simulink library "mttlib"  (R2023a)
settings: Solver=VariableStepAuto  StartTime=0.0  StopTime=10.0  RelTol=1e-3
libraries: simulink x37, etargetslib x17, instrumentseriallib x2
settings Model: Creator=chrismailer  LastModifiedBy=JesseJabezArendse
settings ModelReferenceCC: EnableRefExpFcnMdlSchedulingChecks=on

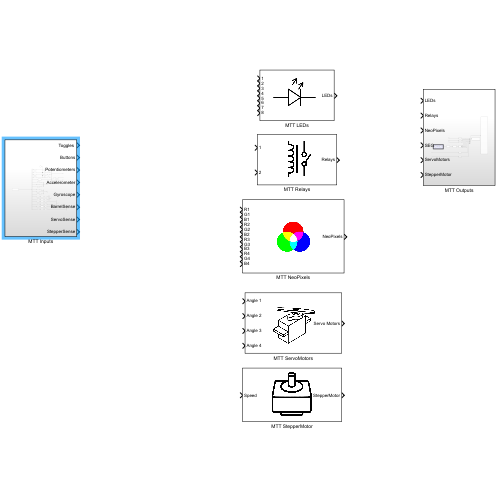
[thumbnail: Simulink's stored preview of the top-level diagram]
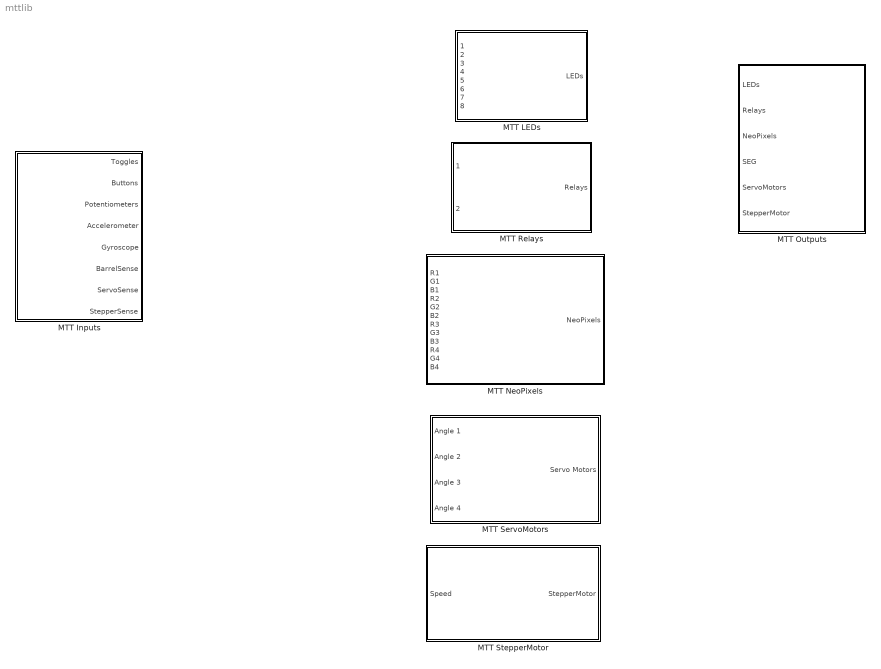
== system mttlib ==
  MTT Inputs : Subsystem
  MTT LEDs : Subsystem
      mask DialogControl DescGroupVar Prompt: MTT LEDs
      mask DialogControl DescTextVar Prompt: Initializing block for using the LEDs on the MTT board.
      mask Display: image('$imagefile'); % Use "Edit Image" on toolstrip to change.
  MTT NeoPixels : Subsystem
      mask DialogControl DescGroupVar Prompt: MTT NeoPixels
      mask DialogControl DescTextVar Prompt: Initializing block for using the NeoPixels on the MTT board.
      mask DialogControl Control2 Prompt: NeoPixels will not shine brigher when using values above 255, the brightness of each colour has been limited for eye comfort.
      mask Display: image('$imagefile'); % Use "Edit Image" on toolstrip to change.
  MTT Outputs : Subsystem
  MTT Relays : Subsystem
      mask DialogControl Container1 Prompt: MTT Relays
      mask DialogControl Control1 Prompt: Initializing block for the Relays on the MTT board.
      mask Display: image('$imagefile'); % Use "Edit Image" on toolstrip to change.
  MTT ServoMotors : Subsystem  mask{maxAngle1=0, startingTime1=0, maxAngle2=0, startingTime2=0, maxAngle3=0, startingTime3=0, maxAngle4=0, startingTime4=0}
      mask prompts: maxAngle1 "Max Angle (°):"; startingTime1 "Starting Time (μs):"; maxAngle2 "Max Angle (°):"; startingTime2 "Starting Time (μs):"; maxAngle3 "Max Angle (°):"; startingTime3 "Starting Time (μs):"; maxAngle4 "Max Angle (°):"; startingTime4 "Starting Time (μs):"
      mask DialogControl DescGroupVar Prompt: MTT ServoMotors
      mask DialogControl DescTextVar Prompt: Initializing block to use Servo Motors with MTT Board.
      mask DialogControl Control2 Prompt: Make sure to use non-zero values for servo parameters, they will not function otherwise.
      mask DialogControl Container1 Prompt: ServoMotor 1
      mask DialogControl Container2 Prompt: ServoMotor 2
      mask DialogControl Container3 Prompt: ServoMotor 3
      mask DialogControl Container4 Prompt: ServoMotor 4
      mask Display: image('$imagefile'); % Use "Edit Image" on toolstrip to change.
  MTT StepperMotor : Subsystem  mask{stepperMode=Full, stepperRevolution=1024}
      mask prompts: stepperMode "Mode:"; stepperRevolution "No. of steps for revolution:"
      mask TypeOptions stepperMode: Full | Wave | Half
      mask DialogControl DescGroupVar Prompt: MTT StepperMotor
      mask DialogControl DescTextVar Prompt: Initializing block for using a Stepper Motor on the MTT board.
      mask Display: image('$imagefile'); % Use "Edit Image" on toolstrip to change.

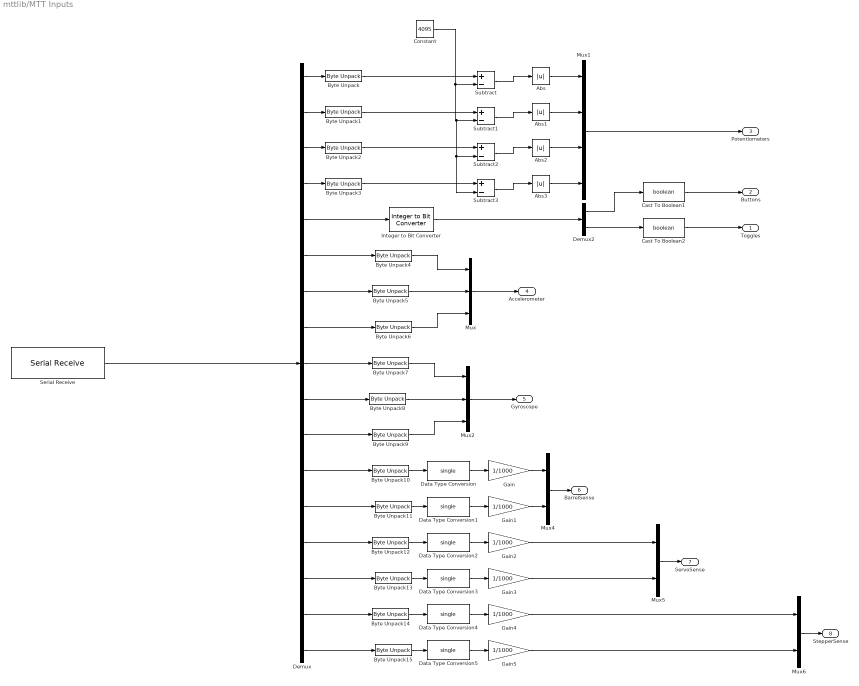
== system mttlib/MTT Inputs ==
  Abs{,1..3} (4 alike) : Abs  SaturateOnIntegerOverflow=off
  Byte Unpack{,1..3} (4 alike) : etargetslib/Byte Unpack  dimensions={[1]}  datatypes={'uint16'}  byteAlign=1
  Byte Unpack{10..15} (6 alike) : etargetslib/Byte Unpack  dimensions={[1]}  datatypes={'int16'}  byteAlign=1
  Byte Unpack{4..9} (6 alike) : etargetslib/Byte Unpack  dimensions={[1]}  datatypes={'single'}  byteAlign=1
  Cast To Boolean1 : DataTypeConversion  OutDataTypeStr=boolean  SaturateOnIntegerOverflow=off  RndMeth=Floor
  Cast To Boolean2 : DataTypeConversion  OutDataTypeStr=boolean  SaturateOnIntegerOverflow=off  RndMeth=Floor
  Constant : Constant  Value=4095
  Data Type Conversion{,1..5} (6 alike) : DataTypeConversion  OutDataTypeStr=single  SaturateOnIntegerOverflow=off  RndMeth=Floor
  Demux : Demux  Outputs=[2,2,2,2,1,4,4,4,4,4,4,2,2,2,2,2,2]
  Demux2 : Demux  Outputs=2
  Gain{,1..5} (6 alike) : Gain  Gain=1/1000
  Integer to Bit Converter : simulink/Logic and Bit Operations/Integer to Bit Converter  nbits=8  signedInputValues=Unsigned  bitOrder=MSB first  outDtype=boolean
  Mux : Mux  Inputs=3
  Mux1 : Mux
  Mux2 : Mux  Inputs=3
  Mux4 : Mux  Inputs=2
  Mux5 : Mux  Inputs=2
  Mux6 : Mux  Inputs=2
  Serial Receive : instrumentseriallib/Serial Receive  Priority=1  PortSel=COM17  Port=COM17  ComPort=COM17  DataType=uint8  SaveDataType=uint8  ToggleHeader=on  Header=0b10010010  ToggleTerminator=off  Terminator=<none>  CustomTerminator=[]  InputFormat=Column major  ToggleDataSize=on  DataSize=[1 45]  EnableBlockingMode=on  ActionDataUnavailable=Output last received value  ActionWhenDataUnavailable=Output last received value  CustomValue=0  SampleTime=0.01  SimulateUsing=Interpreted execution  BlockInModel=on  aMode=1
  Subtract{,1..3} (4 alike) : Sum  Inputs=+-
  "Toggles " : Outport
  Buttons : Outport  Port=2
  Potentiometers : Outport  Port=3
  Accelerometer : Outport  Port=4
  Gyroscope : Outport  Port=5
  BarrelSense : Outport  Port=6
  ServoSense : Outport  Port=7
  StepperSense : Outport  Port=8
  wires:
  Demux/2 -> Byte Unpack1/1
  Demux2/2 -> Cast To Boolean2/1
  Demux2/1 -> Cast To Boolean1/1
  Integer to Bit Converter/1 -> Demux2/1
  Demux/3 -> Byte Unpack2/1
  Demux/1 -> Byte Unpack/1
  Demux/4 -> Byte Unpack3/1
  Demux/5 -> Integer to Bit Converter/1
  Serial Receive/1 -> Demux/1
  Demux/6 -> Byte Unpack4/1
  Demux/7 -> Byte Unpack5/1
  Demux/8 -> Byte Unpack6/1
  Byte Unpack4/1 -> Mux/1
  Byte Unpack5/1 -> Mux/2
  Byte Unpack6/1 -> Mux/3
  Mux/1 -> Accelerometer/1
  Mux2/1 -> Gyroscope/1
  Demux/11 -> Byte Unpack9/1
  Byte Unpack7/1 -> Mux2/1
  Byte Unpack9/1 -> Mux2/3
  Demux/9 -> Byte Unpack7/1
  Demux/10 -> Byte Unpack8/1
  Byte Unpack8/1 -> Mux2/2
  Demux/12 -> Byte Unpack10/1
  Byte Unpack10/1 -> Data Type Conversion/1
  Demux/13 -> Byte Unpack11/1
  Demux/14 -> Byte Unpack12/1
  Demux/15 -> Byte Unpack13/1
  Demux/16 -> Byte Unpack14/1
  Demux/17 -> Byte Unpack15/1
  Mux4/1 -> BarrelSense/1
  Mux5/1 -> ServoSense/1
  Mux6/1 -> StepperSense/1
  Data Type Conversion/1 -> Gain/1
  Gain/1 -> Mux4/1
  Data Type Conversion1/1 -> Gain1/1
  Byte Unpack11/1 -> Data Type Conversion1/1
  Gain1/1 -> Mux4/2
  Data Type Conversion2/1 -> Gain2/1
  Byte Unpack12/1 -> Data Type Conversion2/1
  Gain2/1 -> Mux5/1
  Data Type Conversion3/1 -> Gain3/1
  Gain3/1 -> Mux5/2
  Data Type Conversion4/1 -> Gain4/1
  Data Type Conversion5/1 -> Gain5/1
  Byte Unpack14/1 -> Data Type Conversion4/1
  Byte Unpack13/1 -> Data Type Conversion3/1
  Byte Unpack15/1 -> Data Type Conversion5/1
  Gain4/1 -> Mux6/1
  Gain5/1 -> Mux6/2
  Mux1/1 -> Potentiometers/1
  Cast To Boolean1/1 -> Buttons/1
  Cast To Boolean2/1 -> "Toggles "/1
  Abs/1 -> Mux1/1
  Abs1/1 -> Mux1/2
  Abs2/1 -> Mux1/3
  Abs3/1 -> Mux1/4
  Subtract/1 -> Abs/1
  Byte Unpack/1 -> Subtract/1
  Subtract1/1 -> Abs1/1
  Byte Unpack1/1 -> Subtract1/1
  Subtract2/1 -> Abs2/1
  Byte Unpack2/1 -> Subtract2/1
  Subtract3/1 -> Abs3/1
  Byte Unpack3/1 -> Subtract3/1
  Constant/1 -> Subtract3/2, Subtract2/2, Subtract1/2, Subtract/2

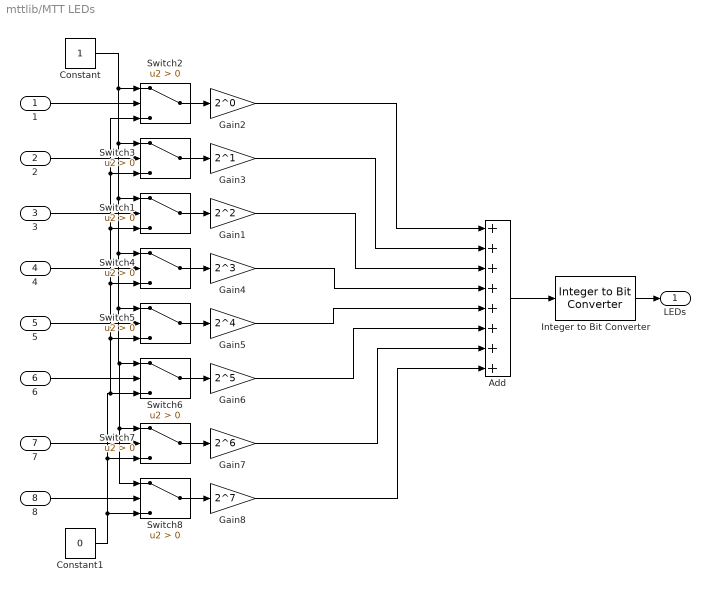
== system mttlib/MTT LEDs ==
  1 : Inport
  2 : Inport  Port=2
  3 : Inport  Port=3
  4 : Inport  Port=4
  5 : Inport  Port=5
  6 : Inport  Port=6
  7 : Inport  Port=7
  8 : Inport  Port=8
  Add : Sum  Inputs=++++++++
  Constant : Constant
  Constant1 : Constant  Value=0
  Gain1 : Gain  Gain=2^2
  Gain2 : Gain  Gain=2^0
  Gain3 : Gain  Gain=2^1
  Gain4 : Gain  Gain=2^3
  Gain5 : Gain  Gain=2^4
  Gain6 : Gain  Gain=2^5
  Gain7 : Gain  Gain=2^6
  Gain8 : Gain  Gain=2^7
  Integer to Bit Converter : simulink/Logic and Bit Operations/Integer to Bit Converter  nbits=8  signedInputValues=Unsigned  bitOrder=MSB first  outDtype=Inherit via internal rule
  Switch{1..8} (8 alike) : Switch  Criteria=u2 > Threshold  SaturateOnIntegerOverflow=off  InputSameDT=off
  LEDs : Outport
  wires:
  Add/1 -> Integer to Bit Converter/1
  Integer to Bit Converter/1 -> LEDs/1
  1/1 -> Switch2/2
  Switch2/1 -> Gain2/1
  2/1 -> Switch3/2
  Switch3/1 -> Gain3/1
  3/1 -> Switch1/2
  Switch1/1 -> Gain1/1
  4/1 -> Switch4/2
  Switch4/1 -> Gain4/1
  5/1 -> Switch5/2
  Switch5/1 -> Gain5/1
  6/1 -> Switch6/2
  Switch6/1 -> Gain6/1
  7/1 -> Switch7/2
  Switch7/1 -> Gain7/1
  8/1 -> Switch8/2
  Switch8/1 -> Gain8/1
  Constant/1 -> Switch8/1, Switch7/1, Switch6/1, Switch5/1, Switch4/1, Switch1/1, Switch3/1, Switch2/1
  Constant1/1 -> Switch8/3, Switch3/3, Switch2/3, Switch1/3, Switch4/3, Switch5/3, Switch6/3, Switch7/3
  Gain2/1 -> Add/1
  Gain3/1 -> Add/2
  Gain1/1 -> Add/3
  Gain4/1 -> Add/4
  Gain5/1 -> Add/5
  Gain6/1 -> Add/6
  Gain7/1 -> Add/7
  Gain8/1 -> Add/8

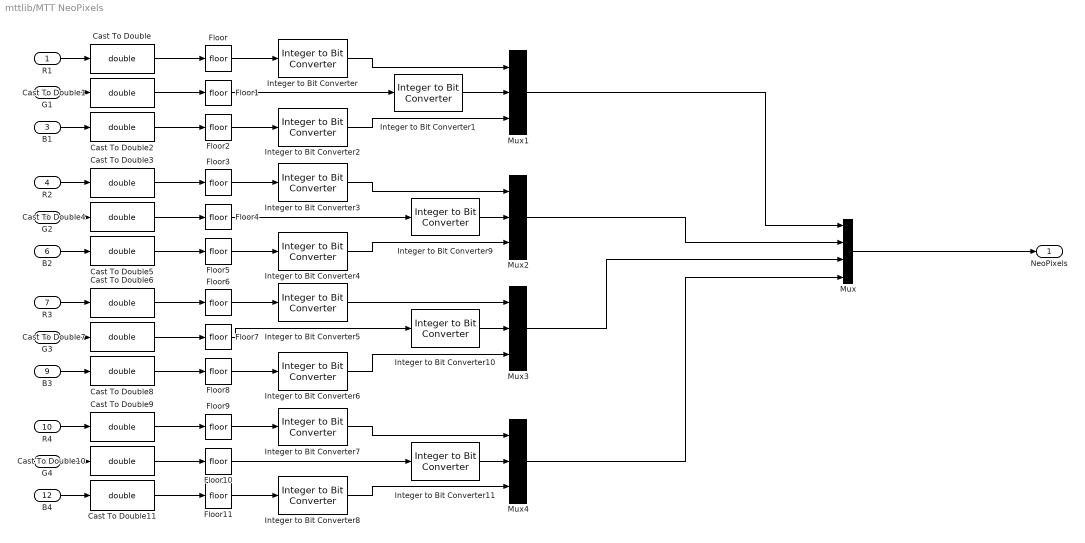
== system mttlib/MTT NeoPixels ==
  R1 : Inport
  G1 : Inport  Port=2
  B1 : Inport  Port=3
  R2 : Inport  Port=4
  G2 : Inport  Port=5
  B2 : Inport  Port=6
  R3 : Inport  Port=7
  G3 : Inport  Port=8
  B3 : Inport  Port=9
  R4 : Inport  Port=10
  G4 : Inport  Port=11
  B4 : Inport  Port=12
  Cast To Double{,1..11} (12 alike) : DataTypeConversion  OutDataTypeStr=double  SaturateOnIntegerOverflow=off  RndMeth=Floor
  Floor{,1..11} (12 alike) : Rounding
  Integer to Bit Converter{,1..11} (12 alike) : simulink/Logic and Bit Operations/Integer to Bit Converter  nbits=8  signedInputValues=Unsigned  bitOrder=MSB first  outDtype=Inherit via internal rule
  Mux : Mux
  Mux{1..4} (4 alike) : Mux  Inputs=3
  NeoPixels : Outport
  wires:
  Mux/1 -> NeoPixels/1
  G1/1 -> Cast To Double1/1
  R1/1 -> Cast To Double/1
  B1/1 -> Cast To Double2/1
  B2/1 -> Cast To Double5/1
  R2/1 -> Cast To Double3/1
  G2/1 -> Cast To Double4/1
  B3/1 -> Cast To Double8/1
  R3/1 -> Cast To Double6/1
  G3/1 -> Cast To Double7/1
  B4/1 -> Cast To Double11/1
  R4/1 -> Cast To Double9/1
  G4/1 -> Cast To Double10/1
  Mux4/1 -> Mux/4
  Mux3/1 -> Mux/3
  Mux2/1 -> Mux/2
  Mux1/1 -> Mux/1
  Integer to Bit Converter/1 -> Mux1/1
  Integer to Bit Converter1/1 -> Mux1/2
  Integer to Bit Converter2/1 -> Mux1/3
  Integer to Bit Converter3/1 -> Mux2/1
  Integer to Bit Converter4/1 -> Mux2/3
  Integer to Bit Converter5/1 -> Mux3/1
  Integer to Bit Converter6/1 -> Mux3/3
  Integer to Bit Converter7/1 -> Mux4/1
  Integer to Bit Converter8/1 -> Mux4/3
  Integer to Bit Converter9/1 -> Mux2/2
  Integer to Bit Converter10/1 -> Mux3/2
  Integer to Bit Converter11/1 -> Mux4/2
  Floor/1 -> Integer to Bit Converter/1
  Cast To Double/1 -> Floor/1
  Cast To Double1/1 -> Floor1/1
  Cast To Double2/1 -> Floor2/1
  Cast To Double3/1 -> Floor3/1
  Cast To Double4/1 -> Floor4/1
  Cast To Double5/1 -> Floor5/1
  Cast To Double6/1 -> Floor6/1
  Cast To Double7/1 -> Floor7/1
  Cast To Double8/1 -> Floor8/1
  Cast To Double9/1 -> Floor9/1
  Cast To Double10/1 -> Floor10/1
  Cast To Double11/1 -> Floor11/1
  Floor1/1 -> Integer to Bit Converter1/1
  Floor2/1 -> Integer to Bit Converter2/1
  Floor3/1 -> Integer to Bit Converter3/1
  Floor4/1 -> Integer to Bit Converter9/1
  Floor5/1 -> Integer to Bit Converter4/1
  Floor6/1 -> Integer to Bit Converter5/1
  Floor7/1 -> Integer to Bit Converter10/1
  Floor8/1 -> Integer to Bit Converter6/1
  Floor9/1 -> Integer to Bit Converter7/1
  Floor10/1 -> Integer to Bit Converter11/1
  Floor11/1 -> Integer to Bit Converter8/1

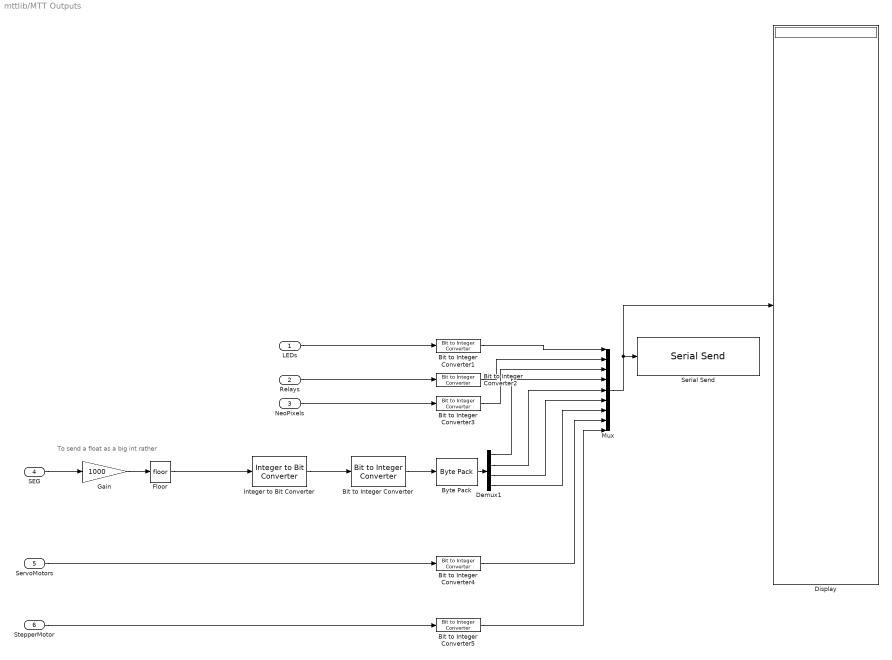
== system mttlib/MTT Outputs ==
  note: To send a float as a big int rather
  LEDs : Inport
  Relays : Inport  Port=2
  NeoPixels : Inport  Port=3
  SEG : Inport  Port=4
  ServoMotors : Inport  Port=5
  StepperMotor : Inport  Port=6
  Bit to Integer Converter : simulink/Logic and Bit Operations/Bit to Integer Converter  nbits=32  bitOrder=MSB first  signedOutputValues=Unsigned  outDtype=int32  outDtypeSigned=Inherit via internal rule
  Bit to Integer Converter{1..5} (5 alike) : simulink/Logic and Bit Operations/Bit to Integer Converter  nbits=8  bitOrder=MSB first  signedOutputValues=Unsigned  outDtype=uint8  outDtypeSigned=Inherit via internal rule
  Byte Pack : etargetslib/Byte Pack  datatypes={'int32'}  byteAlign=1
  Demux1 : Demux
  Display : Display
  Floor : Rounding
  Gain : Gain  Gain=1000
  Integer to Bit Converter : simulink/Logic and Bit Operations/Integer to Bit Converter  nbits=32  signedInputValues=Signed  bitOrder=MSB first  outDtype=Inherit via internal rule
  Mux : Mux  Inputs=9
  Serial Send : instrumentseriallib/Serial Send  Priority=1  PortSel=COM17  Port=COM17  ComPort=COM17  Header=[0b10010010 0b01001001]  Terminator=<none>  CustomTerminator=[]  EnableBlockingMode=on  SimulateUsing=Interpreted execution  BlockInModel=on  aMode=1
  wires:
  Demux1/1 -> Mux/4
  Bit to Integer Converter/1 -> Byte Pack/1
  Bit to Integer Converter3/1 -> Mux/3
  Bit to Integer Converter2/1 -> Mux/2
  SEG/1 -> Gain/1
  Demux1/2 -> Mux/5
  LEDs/1 -> Bit to Integer Converter1/1
  Bit to Integer Converter1/1 -> Mux/1
  Byte Pack/1 -> Demux1/1
  Relays/1 -> Bit to Integer Converter2/1
  NeoPixels/1 -> Bit to Integer Converter3/1
  Gain/1 -> Floor/1
  Floor/1 -> Integer to Bit Converter/1
  Integer to Bit Converter/1 -> Bit to Integer Converter/1
  Demux1/3 -> Mux/6
  Demux1/4 -> Mux/7
  Mux/1 -> Display/1, Serial Send/1
  ServoMotors/1 -> Bit to Integer Converter4/1
  Bit to Integer Converter4/1 -> Mux/8
  StepperMotor/1 -> Bit to Integer Converter5/1
  Bit to Integer Converter5/1 -> Mux/9

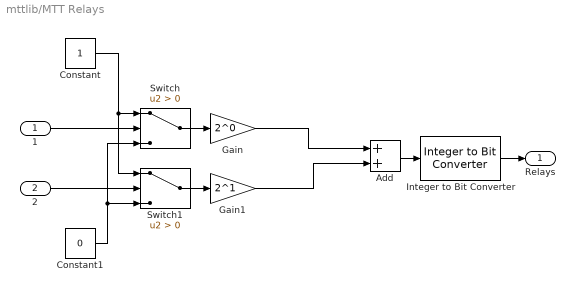
== system mttlib/MTT Relays ==
  1 : Inport
  2 : Inport  Port=2
  Add : Sum
  Constant : Constant
  Constant1 : Constant  Value=0
  Gain : Gain  Gain=2^0
  Gain1 : Gain  Gain=2^1
  Integer to Bit Converter : simulink/Logic and Bit Operations/Integer to Bit Converter  nbits=8  signedInputValues=Unsigned  bitOrder=MSB first  outDtype=Inherit via internal rule
  Switch : Switch  Criteria=u2 > Threshold  SaturateOnIntegerOverflow=off  InputSameDT=off
  Switch1 : Switch  Criteria=u2 > Threshold  SaturateOnIntegerOverflow=off  InputSameDT=off
  Relays : Outport
  wires:
  Constant/1 -> Switch1/1, Switch/1
  Constant1/1 -> Switch1/3, Switch/3
  1/1 -> Switch/2
  2/1 -> Switch1/2
  Integer to Bit Converter/1 -> Relays/1
  Switch/1 -> Gain/1
  Switch1/1 -> Gain1/1
  Add/1 -> Integer to Bit Converter/1
  Gain/1 -> Add/1
  Gain1/1 -> Add/2

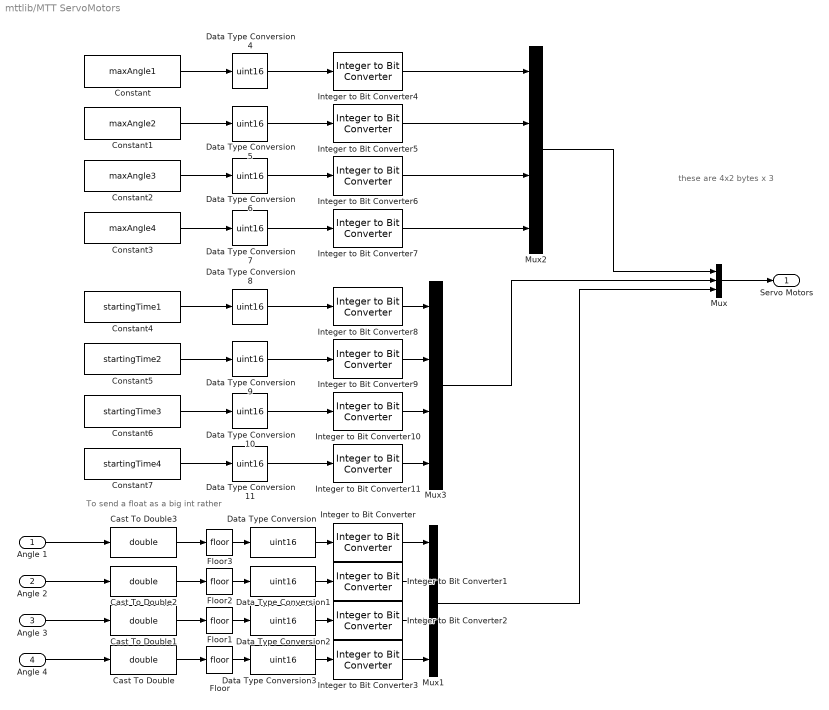
== system mttlib/MTT ServoMotors ==
  note: these are 4x2 bytes x 3
  note: To send a float as a big int rather
  Angle 1 : Inport
  Angle 2 : Inport  Port=2
  Angle 3 : Inport  Port=3
  Angle 4 : Inport  Port=4
  Cast To Double{,1..3} (4 alike) : DataTypeConversion  OutDataTypeStr=double  SaturateOnIntegerOverflow=off  RndMeth=Floor
  Constant : Constant  Value=maxAngle1  OutDataTypeStr=uint16
  Constant1 : Constant  Value=maxAngle2
  Constant2 : Constant  Value=maxAngle3
  Constant3 : Constant  Value=maxAngle4
  Constant4 : Constant  Value=startingTime1
  Constant5 : Constant  Value=startingTime2
  Constant6 : Constant  Value=startingTime3
  Constant7 : Constant  Value=startingTime4
  Data Type Conversion{,1..3} (4 alike) : DataTypeConversion  OutDataTypeStr=uint16  SaturateOnIntegerOverflow=off  RndMeth=Floor
  Data Type Conversion{4..11} (8 alike) : DataTypeConversion  OutDataTypeStr=uint16  RndMeth=Nearest  SaturateOnIntegerOverflow=off
  Floor{,1..3} (4 alike) : Rounding
  Integer to Bit Converter{,1..11} (12 alike) : simulink/Logic and Bit Operations/Integer to Bit Converter  nbits=16  signedInputValues=Unsigned  bitOrder=MSB first  outDtype=Inherit via internal rule
  Mux : Mux  Inputs=3
  Mux1 : Mux
  Mux2 : Mux
  Mux3 : Mux
  Servo Motors : Outport
  wires:
  Mux/1 -> Servo Motors/1
  Constant/1 -> Data Type Conversion4/1
  Constant1/1 -> Data Type Conversion5/1
  Constant2/1 -> Data Type Conversion6/1
  Constant3/1 -> Data Type Conversion7/1
  Constant4/1 -> Data Type Conversion8/1
  Constant6/1 -> Data Type Conversion10/1
  Constant7/1 -> Data Type Conversion11/1
  Constant5/1 -> Data Type Conversion9/1
  Mux1/1 -> Mux/3
  Mux3/1 -> Mux/2
  Mux2/1 -> Mux/1
  Angle 4/1 -> Cast To Double/1
  Cast To Double/1 -> Floor/1
  Cast To Double1/1 -> Floor1/1
  Angle 3/1 -> Cast To Double1/1
  Cast To Double2/1 -> Floor2/1
  Angle 2/1 -> Cast To Double2/1
  Cast To Double3/1 -> Floor3/1
  Floor3/1 -> Data Type Conversion/1
  Angle 1/1 -> Cast To Double3/1
  Data Type Conversion/1 -> Integer to Bit Converter/1
  Integer to Bit Converter/1 -> Mux1/1
  Data Type Conversion1/1 -> Integer to Bit Converter1/1
  Floor2/1 -> Data Type Conversion1/1
  Integer to Bit Converter1/1 -> Mux1/2
  Data Type Conversion2/1 -> Integer to Bit Converter2/1
  Floor1/1 -> Data Type Conversion2/1
  Integer to Bit Converter2/1 -> Mux1/3
  Data Type Conversion3/1 -> Integer to Bit Converter3/1
  Floor/1 -> Data Type Conversion3/1
  Integer to Bit Converter3/1 -> Mux1/4
  Integer to Bit Converter4/1 -> Mux2/1
  Integer to Bit Converter5/1 -> Mux2/2
  Integer to Bit Converter6/1 -> Mux2/3
  Integer to Bit Converter7/1 -> Mux2/4
  Integer to Bit Converter8/1 -> Mux3/1
  Integer to Bit Converter9/1 -> Mux3/2
  Integer to Bit Converter10/1 -> Mux3/3
  Integer to Bit Converter11/1 -> Mux3/4
  Data Type Conversion4/1 -> Integer to Bit Converter4/1
  Data Type Conversion5/1 -> Integer to Bit Converter5/1
  Data Type Conversion6/1 -> Integer to Bit Converter6/1
  Data Type Conversion7/1 -> Integer to Bit Converter7/1
  Data Type Conversion8/1 -> Integer to Bit Converter8/1
  Data Type Conversion9/1 -> Integer to Bit Converter9/1
  Data Type Conversion10/1 -> Integer to Bit Converter10/1
  Data Type Conversion11/1 -> Integer to Bit Converter11/1

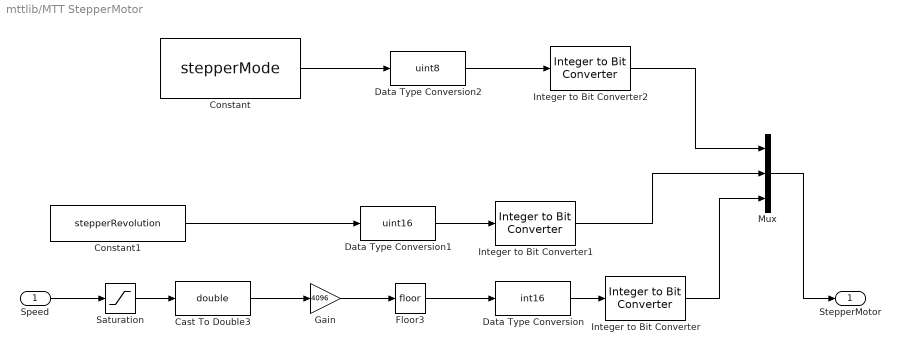
== system mttlib/MTT StepperMotor ==
  Speed : Inport
  Cast To Double3 : DataTypeConversion  OutDataTypeStr=double  SaturateOnIntegerOverflow=off  RndMeth=Floor
  Constant : Constant  Value=stepperMode
  Constant1 : Constant  Value=stepperRevolution
  Data Type Conversion : DataTypeConversion  OutDataTypeStr=int16  SaturateOnIntegerOverflow=off  RndMeth=Floor
  Data Type Conversion1 : DataTypeConversion  OutDataTypeStr=uint16  SaturateOnIntegerOverflow=off  RndMeth=Floor
  Data Type Conversion2 : DataTypeConversion  OutDataTypeStr=uint8  SaturateOnIntegerOverflow=off  RndMeth=Floor
  Floor3 : Rounding
  Gain : Gain  Gain=4096
  Integer to Bit Converter : simulink/Logic and Bit Operations/Integer to Bit Converter  nbits=16  signedInputValues=Signed  bitOrder=MSB first  outDtype=Inherit via internal rule
  Integer to Bit Converter1 : simulink/Logic and Bit Operations/Integer to Bit Converter  nbits=16  signedInputValues=Unsigned  bitOrder=MSB first  outDtype=Inherit via internal rule
  Integer to Bit Converter2 : simulink/Logic and Bit Operations/Integer to Bit Converter  nbits=8  signedInputValues=Unsigned  bitOrder=MSB first  outDtype=Inherit via internal rule
  Mux : Mux  Inputs=3
  Saturation : Saturate  UpperLimit=1000  LowerLimit=-1000
  StepperMotor : Outport
  wires:
  Data Type Conversion/1 -> Integer to Bit Converter/1
  Cast To Double3/1 -> Gain/1
  Speed/1 -> Saturation/1
  Floor3/1 -> Data Type Conversion/1
  Integer to Bit Converter/1 -> Mux/3
  Saturation/1 -> Cast To Double3/1
  Gain/1 -> Floor3/1
  Constant1/1 -> Data Type Conversion1/1
  Data Type Conversion1/1 -> Integer to Bit Converter1/1
  Integer to Bit Converter1/1 -> Mux/2
  Mux/1 -> StepperMotor/1
  Data Type Conversion2/1 -> Integer to Bit Converter2/1
  Constant/1 -> Data Type Conversion2/1
  Integer to Bit Converter2/1 -> Mux/1
